simulink model "CtrlAumPertRampa4"  (R2022b)
settings: Solver=ode45  StartTime=0.0  StopTime=700  RelTol=1e-3  EnableMultiTasking=on
settings Model: Creator=adolfobs  LastModifiedBy=adolfo
settings SolverCC: AlgebraicLoopSolver=TrustRegion
settings DataIOCC: LimitDataPoints=on  MaxDataPoints=25000  SaveFormat=Array  SignalLoggingSaveFormat=ModelDataLogs  ReturnWorkspaceOutputs=off
settings OptimizationCC: BlockReduction=off  BooleanDataType=off  InitFltsAndDblsToZero=on  LifeSpan=inf
settings DebuggingCC: SaveWithParameterizedLinksMsg=none  UnderspecifiedInitializationDetection=Classic  MergeDetectMultiDrivingBlocksExec=none  SignalResolutionControl=TryResolveAllWithWarning  MultiTaskDSMMsg=warning  MultiTaskCondExecSysMsg=none  UnconnectedInputMsg=warning  UnconnectedOutputMsg=warning  UnconnectedLineMsg=warning  SFUnexpectedBacktrackingDiag=warning  SFNoUnconditionalDefaultTransitionDiag=warning  SFExecutionAtInitializationDiag=none  SFMachineParentedDataDiag=warning  ArithmeticOperatorsInVariantConditions=warning
settings HardwareCC: ProdBitPerPointer=32  ProdBitPerSizeT=32  ProdBitPerPtrDiffT=32  ProdLargestAtomicFloat=None  ProdIntDivRoundTo=Undefined  ProdEndianess=Unspecified  ProdWordSize=32  ProdHWDeviceType=32-bit Generic  TargetUnknown=on
settings ModelReferenceCC: EnableRefExpFcnMdlSchedulingChecks=on  PropagateSignalLabelsOutOfModel=off
settings SFSimCC: SimUseLocalCustomCode=off  CustomCodeUndefinedFunction=UseInterfaceOnly
settings RTWCC: RTWUseLocalCustomCode=off
settings CodeAppCC: StateflowObjectComments=on
settings GRTTargetCC: TargetFcnLib=ansi_tfl_tmw.mat  TargetLangStandard=C89/C90 (ANSI)  CombineOutputUpdateFcns=off  GRTInterface=on
settings ConfigComp: CovMetricSettings=dw  CovSaveCumulativeToWorkspaceVar=on  CovSaveSingleToWorkspaceVar=on  CovExternalEMLEnable=off

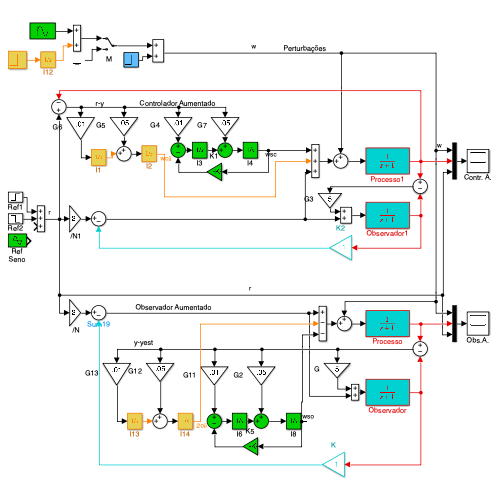
[thumbnail: Simulink's stored preview of the top-level diagram]
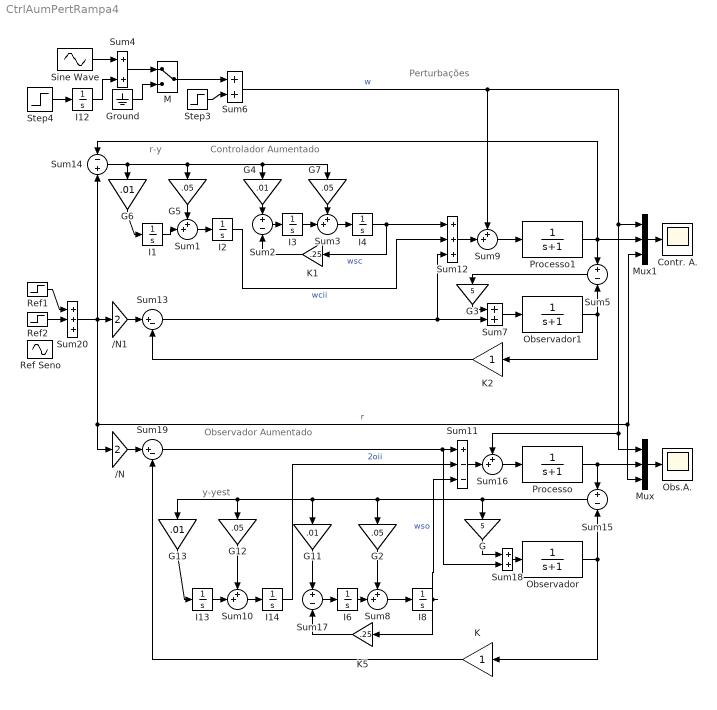
== system CtrlAumPertRampa4 ==
  note: Observador Aumentado
  note: y-yest
  note: r-y
  note: Perturbações
  note: Controlador Aumentado
  " /N" : Gain  Gain=2  SaturateOnIntegerOverflow=on  OutDataTypeStr=Inherit: Same as input  ParamDataTypeStr=Inherit: Same as input
  " /N1" : Gain  Gain=2  SaturateOnIntegerOverflow=on  OutDataTypeStr=Inherit: Same as input  ParamDataTypeStr=Inherit: Same as input
  Contr. A. : Scope
  G : Gain  Gain=5  SaturateOnIntegerOverflow=on  OutDataTypeStr=Inherit: Same as input  ParamDataTypeStr=Inherit: Same as input
  G{4,6,11,13} (4 alike) : Gain  Gain=.01  SaturateOnIntegerOverflow=on  OutDataTypeStr=Inherit: Same as input  ParamDataTypeStr=Inherit: Same as input
  G{2,5,7,12} (4 alike) : Gain  Gain=.05  SaturateOnIntegerOverflow=on  OutDataTypeStr=Inherit: Same as input  ParamDataTypeStr=Inherit: Same as input
  G3 : Gain  Gain=5  SaturateOnIntegerOverflow=on  OutDataTypeStr=Inherit: Same as input  ParamDataTypeStr=Inherit: Same as input
  Ground : Ground
  I{1..4,6,8,12..14} (9 alike) : Integrator
  K : Gain  SaturateOnIntegerOverflow=on  OutDataTypeStr=Inherit: Same as input  ParamDataTypeStr=Inherit: Same as input
  K1 : Gain  Gain=.25  SaturateOnIntegerOverflow=on  OutDataTypeStr=Inherit: Same as input  ParamDataTypeStr=Inherit: Same as input
  K2 : Gain  SaturateOnIntegerOverflow=on  OutDataTypeStr=Inherit: Same as input  ParamDataTypeStr=Inherit: Same as input
  K5 : Gain  Gain=.25  SaturateOnIntegerOverflow=on  OutDataTypeStr=Inherit: Same as input  ParamDataTypeStr=Inherit: Same as input
  M : ManualSwitch
  Mux : Mux  Inputs=3
  Mux1 : Mux  Inputs=3
  Obs.A. : Scope
  Observador : TransferFcn  Denominator=[1 1]
  Observador1 : TransferFcn  Denominator=[1 1]
  Processo : TransferFcn  Denominator=[1 1]
  Processo1 : TransferFcn  Denominator=[1 1]
  Ref Seno : Sin  Amplitude=.5  Frequency=.02
  Ref1 : Step  Time=100
  Ref2 : Step  Time=300  After=-2
  Sine Wave : Sin  Amplitude=.3  Frequency=.5
  Step3 : Step  Time=140  After=.2
  Step4 : Step  Time=400  After=.01
  Sum{1,3,8..10,16} (6 alike) : Sum  Inputs=++|  InputSameDT=on  SaturateOnIntegerOverflow=on  OutDataTypeStr=Inherit: Same as first input
  Sum11 : Sum  Inputs=+--  InputSameDT=on  SaturateOnIntegerOverflow=on  OutDataTypeStr=Inherit: Same as first input
  Sum12 : Sum  Inputs=+++  InputSameDT=on  SaturateOnIntegerOverflow=on  OutDataTypeStr=Inherit: Same as first input
  Sum13 : Sum  Inputs=|+-  InputSameDT=on  SaturateOnIntegerOverflow=on  OutDataTypeStr=Inherit: Same as first input
  Sum14 : Sum  Inputs=-+  InputSameDT=on  SaturateOnIntegerOverflow=on  OutDataTypeStr=Inherit: Same as first input
  Sum15 : Sum  Inputs=+|-  InputSameDT=on  SaturateOnIntegerOverflow=on  OutDataTypeStr=Inherit: Same as first input
  Sum17 : Sum  Inputs=+|-  InputSameDT=on  SaturateOnIntegerOverflow=on  OutDataTypeStr=Inherit: Same as first input
  Sum{4,6..7,18} (4 alike) : Sum  InputSameDT=on  SaturateOnIntegerOverflow=on  OutDataTypeStr=Inherit: Same as first input
  Sum19 : Sum  Inputs=|+-  InputSameDT=on  SaturateOnIntegerOverflow=on  OutDataTypeStr=Inherit: Same as first input
  Sum2 : Sum  Inputs=+|-  InputSameDT=on  SaturateOnIntegerOverflow=on  OutDataTypeStr=Inherit: Same as first input
  Sum20 : Sum  Inputs=+++  InputSameDT=on  SaturateOnIntegerOverflow=on  OutDataTypeStr=Inherit: Same as first input
  Sum5 : Sum  Inputs=+-  InputSameDT=on  SaturateOnIntegerOverflow=on  OutDataTypeStr=Inherit: Same as first input
  wires:
  Sum9/1 -> Processo1/1
  Sum12/1 -> Sum9/2
  Mux1/1 -> Contr. A./1
  Processo1/1 -> Sum5/1, Sum14/1, Mux1/2
  Step4/1 -> I12/1
  Sum16/1 -> Processo/1
  Mux/1 -> Obs.A./1
  Sum15/1 -> G2/1, G13/1, G12/1, G11/1, G/1
  Sum17/1 -> I6/1
  Observador/1 -> K/1, Sum15/2
  Sum18/1 -> Observador/1
  G/1 -> Sum18/1
  G11/1 -> Sum17/1
  K/1 -> Sum19/2
  Processo/1 -> Sum15/1, Mux/2
  Sum20/1 -> Sum14/2, " /N1"/1, Mux1/3, Mux/3, " /N"/1  "r"
  Sum6/1 -> Sum9/1, Sum16/1, Mux/1, Mux1/1  "w"
  G12/1 -> Sum10/1
  G13/1 -> I13/1
  I14/1 -> Sum11/2  "2oii"
  K5/1 -> Sum17/2
  I12/1 -> Sum4/2
  Sine Wave/1 -> Sum4/1
  Sum4/1 -> M/1
  Ground/1 -> M/2
  G2/1 -> Sum8/1
  Sum8/1 -> I8/1
  I6/1 -> Sum8/2
  I13/1 -> Sum10/2
  Sum10/1 -> I14/1
  Sum13/1 -> Sum12/3, Sum7/2
  Sum5/1 -> G3/1
  Observador1/1 -> K2/1, Sum5/2
  Sum7/1 -> Observador1/1
  G3/1 -> Sum7/1
  K2/1 -> Sum13/2
  " /N1"/1 -> Sum13/1
  I4/1 -> K1/1, Sum12/1  "wsc"
  I8/1 -> K5/1, Sum11/3  "wso"
  Sum14/1 -> G7/1, G4/1, G5/1, G6/1
  Sum2/1 -> I3/1
  G4/1 -> Sum2/1
  G5/1 -> Sum1/1
  G6/1 -> I1/1
  K1/1 -> Sum2/2
  G7/1 -> Sum3/1
  Sum3/1 -> I4/1
  I3/1 -> Sum3/2
  I1/1 -> Sum1/2
  Sum1/1 -> I2/1
  Ref1/1 -> Sum20/1
  I2/1 -> Sum12/2  "wcii"
  Ref2/1 -> Sum20/2
  Sum11/1 -> Sum16/2
  " /N"/1 -> Sum19/1
  M/1 -> Sum6/1
  Step3/1 -> Sum6/2
  Sum19/1 -> Sum18/2, Sum11/1
